simulink model "test_RehaMove3_Simulink2014b"  (R2014b)
settings: Solver=FixedStepDiscrete  SolverMode=SingleTasking  StartTime=0.0  StopTime=inf  FixedStep=0.04  RelTol=1e-3
libraries: simulink x2, LIB_RehaMove3 x1
settings Model: SimulationMode=external  ExtModeTrigDuration=10000  Creator=constantin  LastModifiedBy=valtin
settings OptimizationCC: ExpressionDepthLimit=2147483647  OptimizeModelRefInitCode=on  LifeSpan=1
settings DebuggingCC: UnderspecifiedInitializationDetection=Classic  MergeDetectMultiDrivingBlocksExec=none  FrameProcessingCompatibilityMsg=error  StateNameClashWarn=warning
settings SFSimCC: SimCustomHeaderCode="#include \"rehamove.hpp\""
settings SFSimCC: SimUserIncludeDirs=|
  | /Users/constantin/Documents/retrainer/retrainer.repo/code/trunk/incl/rehamove/
  | /Users/constantin/Documents/retrainer/retrainer.repo/code/trunk/incl/
settings RTWCC: SystemTargetFile=ert_linux.tlc  MakeCommand=make_rtw OPTS=-DWITH_HW OPTIMIZATION_FLAGS=-O3  TemplateMakefile=ert_linux.tmf  Description=Linux Embedded Coder  TargetLang=C++
settings CodeAppCC: IgnoreCustomStorageClasses=off  CustomSymbolStrType=$N$R$M  InternalIdentifier=Classic
settings STFCustomTargetCC: ModelReferenceCompliant=off  GeneratePreprocessorConditionals=Disable all  CombineOutputUpdateFcns=on  ERTCustomFileBanners=on  SupportComplex=off  SupportVariableSizeSignals=on  MATLABClassNameForMDSCustomization=Simulink.SoftwareTarget.ERTCustomization  GRTInterface=off  SystemTargetFile=ert_linux.tlc
settings ERTTargetCC: ModelReferenceCompliant=off  ParMdlRefBuildCompliant=off  CompOptLevelCompliant=off  ConcurrentExecutionCompliant=off  GeneratePreprocessorConditionals=Disable all  ERTFirstTimeCompliant=off  SupportComplex=off  SupportContinuousTime=on  SupportNonInlinedSFcns=on  SupportVariableSizeSignals=on  ModelStepFunctionPrototypeControlCompliant=off  CPPClassGenCompliant=off  ExtMode=on  MultiInstanceErrorCode=None  ERTCustomFileTemplate=ert_linux_file_process.tlc

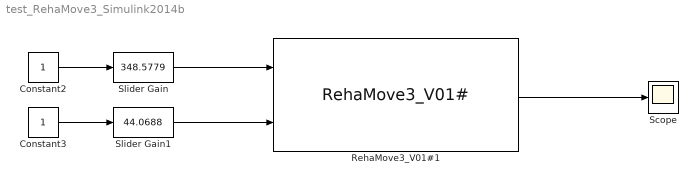
== system test_RehaMove3_Simulink2014b ==
  Constant2 : Constant  OutDataTypeStr=double  SampleTime=0.04
  Constant3 : Constant  OutDataTypeStr=double  SampleTime=0.04
  RehaMove3_V01#1 : LIB_RehaMove3/RehaMove3_V01#  stimDevicePath=/dev/ttyUSB0  stimChannels=[ 1 ]  stimFrequency=25  stimRehaMoveProProtocol="Use the LowLevel protocol   -> Each stimulation pulse is send separatly."  stimMaxCurrent=90  stimMaxPulsWidth=500  stimBlockID=STIM1  stimTextSampleTime=0.04s (based on stimulation frequency)  SampleTime=0.04  stimThreadInit=on  stimThreadData=on  stimAbortError=1  stimTestAgain=2  llPulseShape=0  llNumberOfParts=1  llMaxStimVoltage=90V  llActivateDenervation=off  Parameter58=0  miscPrintBlockParam=off  miscPrintDeviceInfos=off  miscPrintSendInfos=off  miscPrintReceiveInfos=off  miscPrintInitInfos=off  miscPrintStimInfos=off  miscPrintRMPInitSettings=on  miscPrintSequenceErrors=on  miscPrintCorrectionChargeWarnings=on  miscPrintStats=on  miscUseColors=on  miscEnableAdvancedSettings=off  miscDisableVersionCheck=off
  Scope : Scope
      settings: TimeRange=auto  LimitDataPoints=on  MaxDataPoints=5000  SaveToWorkspace=off  SaveName=ScopeData  YMin=-10  YMax=10  SampleTime=-1  DataFormat=Array
  Slider Gain : simulink/Math Operations/Slider Gain  low=0  gain=348.5779  high=510
  Slider Gain1 : simulink/Math Operations/Slider Gain  low=0  gain=44.0688  high=130
  wires:
  RehaMove3_V01#1/1 -> Scope/1
  Slider Gain/1 -> RehaMove3_V01#1/1
  Slider Gain1/1 -> RehaMove3_V01#1/2
  Constant2/1 -> Slider Gain/1
  Constant3/1 -> Slider Gain1/1
